simulink model "HSM_SMC_Final"  (R2018a)
settings: Solver=VariableStepAuto  StartTime=0.0  StopTime=0.1  RelTol=1e-3
InitFcn:
  | fsw = 20e3;
  | T = 1.0/fsw;
  | 
  | J=1.2e-7;
  | Pp = 50;
  | Ls=4.2e-3;
  | Rs=2.1;
  | Flux = 0.00425; %(Vs)
  | Km=Pp*Flux;
  | T_detent = 0.00065; %Nm
  | %------------------------------------
  | Ti=Ls/Rs;
  | rpmmax=200.0;
  | Tn = 2.0/100; %rated torque-Nm
  | TL = Tn;
  | Vdc = 24; %Vdc
  | umax=24; %dien ap cuc dai
  | imax=6; %dong cuc dai cua dong co
  | %------------------------------------
  | %Current controller
  | Kp_idq=0.5*umax/imax;
  | Ti_idq = Ls/Rs;
  | %Ti_idq = 0.009;
  | Ki_idq = Kp_idq/Ti_idq;
  | 
  | %Speed controller
  | Kp_Speed=imax/rpmmax;
  | Ti_Speed=0.25;
  | Ki_Speed = Kp_Speed/Ti_Speed;
  | T_spd = 1/1000;
  | 
  | %q axis maximum back EMF
  | EMFd_max  = (rpmmax/9.55)*Pp*Ls*imax;
  | Kp_Posision=rpmmax/(2*pi);
  | 
  | %ESO
  | fo = fsw/20;
  | %wo = 2*pi*fo;
  | wo = 200;
  | Beta1 = 2*wo;
  | Beta2 = wo*wo;
  | 
  | %Luenberger obs
  | K1 = 400;
  | K2 = 40000;
  | 
  | %PLL
  | kp = 6000;
  | ki = 60000;
  | 
  | %SMO
  | Ksw = 500;
  | wc = 2*pi*10;
undefined symbols (not defined in the file or in its folder): sigbuilder_block
libraries: powerlib x11, powerlib_meascontrol x1
settings Model: Creator=Admin  LastModifiedBy=DATPC
settings DataIOCC: ReturnWorkspaceOutputs=on
settings SFSimCC: SimUseLocalCustomCode=on
settings RTWCC: RTWUseLocalCustomCode=on

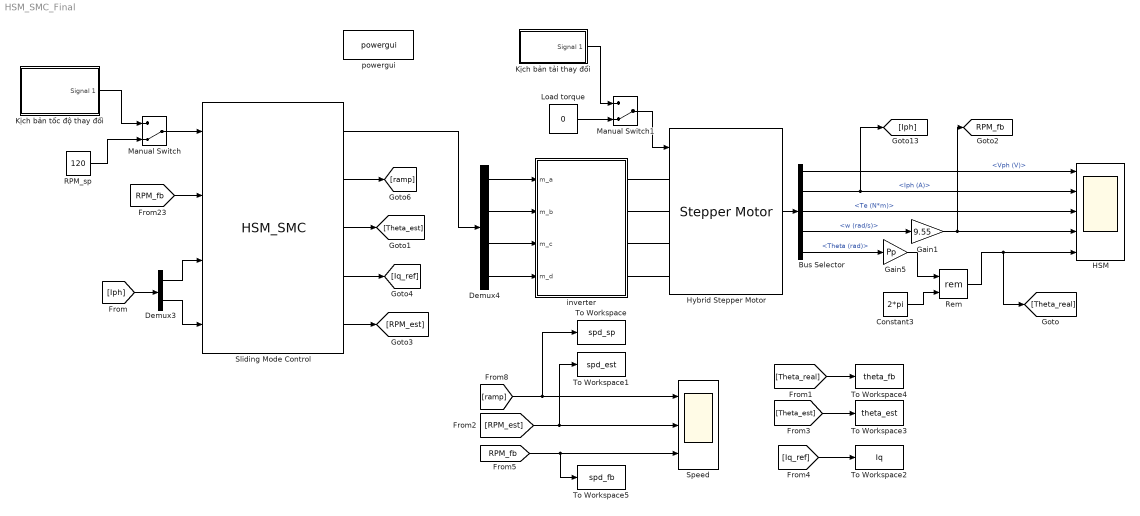
== system HSM_SMC_Final ==
  " Hybrid Stepper Motor" : powerlib/Machines/Stepper Motor  MotorType=Permanent-magnet / Hybrid  NumberOfPhases_1=2  NumberOfPhases_2=3  PresetModel_1=<empty>  PresetModel_2=<empty>  L=4.85e-3  Lmax=10e-3  Lmin=2e-3  R=2.5  Step_angle=1.8  Psim=0.00424  Tdm=0.00065  J=0.00058  B=0.0013  w0=0  pos0=0  TsPowergui=0  TsBlock=-1
      settings: SourceProductBaseCode=PS
  Bus Selector : BusSelector  OutputSignals=Vph (V),Iph (A),Te (N*m),w (rad/s),Theta (rad)
  Constant3 : Constant  Value=2*pi
  Demux3 : Demux  Outputs=2
  Demux4 : Demux
  Gain1 : Gain  Gain=9.55
  Gain5 : Gain  Gain=Pp
  "HSM " : Scope  NumInputPorts=5
  Kịch bản tải thay đổi : Subsystem  Tag=STV Subsys  LoadFcn=sigbuilder_block('load');  StartFcn=sigbuilder_block('start');  StopFcn=sigbuilder_block('stop');  ClipboardFcn=sigbuilder_block('clipboard');  mask(Sigbuilder block){tuvar=[0:10]}
      mask help: Simulink:masks:SigbuilderBlock_MD
      mask init:
      | if ~strcmp(get_param(bdroot(gcbh),'SimulationStatus'),'stopped') tuvar = sigbuilder_block('maskInit'); end
      settings: CopyFcn=sigbuilder_block('copy');  DeleteFcn=sigbuilder_block('delete');  ModelCloseFcn=sigbuilder_block('modelClose');  PreSaveFcn=sigbuilder_block('preSave');  PauseFcn=sigbuilder_block('pause');  ContinueFcn=sigbuilder_block('continue');  NameChangeFcn=sigbuilder_block('namechange');  OpenFcn=sigbuilder_block('open',[69.75 172.5 1141.5 477.75 ]);  CloseFcn=sigbuilder_block('close');
      mask Display: plot(0, 0, 100, 100,[2, 2, 32, 32, 2], [68, 8, 8, 68, 68],[32, 2], [38, 38], [32, 19, 2],[53, 60, 44], [32, 17, 17, 2],[16, 16, 31, 31]);txt = getActiveGroup(gcbh);text(2, 100, txt,'verticalAlignment', 'top');
  Kịch bản tốc độ thay đổi : Subsystem  Tag=STV Subsys  LoadFcn=sigbuilder_block('load');  StartFcn=sigbuilder_block('start');  StopFcn=sigbuilder_block('stop');  ClipboardFcn=sigbuilder_block('clipboard');  mask(Sigbuilder block){tuvar=[0:10]}
      mask help: Simulink:masks:SigbuilderBlock_MD
      mask init:
      | if ~strcmp(get_param(bdroot(gcbh),'SimulationStatus'),'stopped') tuvar = sigbuilder_block('maskInit'); end
      settings: CopyFcn=sigbuilder_block('copy');  DeleteFcn=sigbuilder_block('delete');  ModelCloseFcn=sigbuilder_block('modelClose');  PreSaveFcn=sigbuilder_block('preSave');  PauseFcn=sigbuilder_block('pause');  ContinueFcn=sigbuilder_block('continue');  NameChangeFcn=sigbuilder_block('namechange');  OpenFcn=sigbuilder_block('open',[6 30 1428 681.75 ]);  CloseFcn=sigbuilder_block('close');
      mask Display: plot(0, 0, 100, 100,[2, 2, 32, 32, 2], [68, 8, 8, 68, 68],[32, 2], [38, 38], [32, 19, 2],[53, 60, 44], [32, 17, 17, 2],[16, 16, 31, 31]);txt = getActiveGroup(gcbh);text(2, 100, txt,'verticalAlignment', 'top');
  Load torque : Constant  Value=0
  Manual Switch : ManualSwitch  CurrentSetting=0
  Manual Switch1 : ManualSwitch  CurrentSetting=0
  RPM_sp : Constant  Value=120
  Rem : Math  Operator=rem  SaturateOnIntegerOverflow=on
  Sliding Mode Control : S-Function  InitFcn=try, set_param(gcb,'FunctionName','HSM_SMC'), end  FunctionName=HSM_SMC  SFunctionModules=HSM_SMC_wrapper  SFunctionDeploymentMode=off  EnableBusSupport=off  mask(S-Function Builder){}
      mask help: Simulink:masks:SFunctionBuilder_MD
      mask init:
      | val = [[.9  0.75 0.75 1 1 .9 .9 1]',[1 1 0.75 0.75 .9 .9 1 .9]'];try , sys = get_param(gcb,'SfunBuilderFcnName');if isempty(sys), sys = get_param(gcb,'FunctionName'); end,catch, sys = get_param(gcb,'FunctionName'); end
      settings: CopyFcn=set_param(gcbh,'LinkStatus','none')  PreSaveFcn=try, set_param(gcb,'FunctionName','HSM_SMC'), end  OpenFcn=sfunctionwizard(gcbh)
      mask Display: plot(val(:,1),val(:,2)),disp(sys), port_label('input',1,'RPM_sp'), port_label('input',2,'RPM_fb'), port_label('input',3,'Ia_fb'), port_label('input',4,'Ib_fb'), port_label('output',1,'m'), port_label('output',2,'ramp'), port_label('output',3,'Theta_est'), port_label('output',4,'Iq_sp'), port_label('output',5,'RPM_est')
  Speed : Scope  NumInputPorts=3
  To Workspace : ToWorkspace  VariableName=spd_sp  SaveFormat=Timeseries  SampleTime=-1
  To Workspace1 : ToWorkspace  VariableName=spd_est  SaveFormat=Timeseries  SampleTime=-1
  To Workspace2 : ToWorkspace  VariableName=Iq  SaveFormat=Timeseries  SampleTime=-1
  To Workspace3 : ToWorkspace  VariableName=theta_est  SaveFormat=Timeseries  SampleTime=-1
  To Workspace4 : ToWorkspace  VariableName=theta_fb  SaveFormat=Timeseries  SampleTime=-1
  To Workspace5 : ToWorkspace  VariableName=spd_fb  SaveFormat=Timeseries  SampleTime=-1
  inverter : Subsystem
  powergui : powerlib/powergui  SimulationMode=Discrete  SampleTime=5e-8  frequency=60  Iterations=50  frequencyindice=0  Pbase=100e6  ErrMax=1e-4  UnitsV=kV  UnitsW=MW  buscounter=0  FunctionMessages=off  echomessages=off  EnableUseOfTLC=off  CurrentSourceSwitches=off  DisableSnubberDevices=off  DisableRonSwitches=off  DisableVfSwitches=off  DisplayEquations=off  SolverType=Tustin/Backward Euler (TBE)  Interpol=off  ExternalGateDelay=off  methode=off  Ts=100  x0status=blocks  SPID=off  SwTol=0  HookPort=off  RestoreLinks=warning  ResistiveCurrentMeasurement=off  Frange=[0:2:500]  Ylog=off  Xlog=on  ShowGrid=off  save=off  variable=ZData  structure=0  ZoomFFT=on  StartTime=0.0  cycles=1  DisplayStyle=1  fundamental=60  FreqAxis=off  MaxFrequency=1000  frequencyindicesteady=1  RmsSteady=1  display=off
  tag scope: RPM_fb=global
  wires:
  Bus Selector/2 -> "HSM "/2, [Iph]  "<Iph (A)>"
  Gain1/1 -> "HSM "/4, [RPM_fb]
  " Hybrid Stepper Motor"/1 -> Bus Selector/1
  Bus Selector/5 -> Gain5/1  "<Theta (rad)>"
  Bus Selector/1 -> "HSM "/1  "<Vph (V)>"
  Bus Selector/3 -> "HSM "/3  "<Te (N*m)>"
  Bus Selector/4 -> Gain1/1  "<w (rad/s)>"
  Demux3/1 -> Sliding Mode Control/3
  Demux3/2 -> Sliding Mode Control/4
  [Iph] -> Demux3/1
  Gain5/1 -> Rem/1
  Rem/1 -> [Theta_real], "HSM "/5
  [RPM_fb] -> Sliding Mode Control/2
  Demux4/1 -> inverter/1(m_a)
  Demux4/2 -> inverter/2(m_b)
  Demux4/3 -> inverter/3(m_c)
  Demux4/4 -> inverter/4(m_d)
  Sliding Mode Control/1 -> Demux4/1
  Manual Switch/1 -> Sliding Mode Control/1
  Constant3/1 -> Rem/2
  RPM_sp/1 -> Manual Switch/2
  Kịch bản tốc độ thay đổi/1(Signal 1) -> Manual Switch/1
  Manual Switch1/1 -> " Hybrid Stepper Motor"/1
  Load torque/1 -> Manual Switch1/2
  Kịch bản tải thay đổi/1(Signal 1) -> Manual Switch1/1
  Sliding Mode Control/5 -> [RPM_est]
  [RPM_est] -> To Workspace1/1, Speed/2
  Sliding Mode Control/2 -> [ramp]
  Sliding Mode Control/3 -> [Theta_est]
  Sliding Mode Control/4 -> [Iq_ref]
  [Iq_ref] -> To Workspace2/1
  [Theta_real] -> To Workspace4/1
  [Theta_est] -> To Workspace3/1
  [ramp] -> To Workspace/1, Speed/1
  [RPM_fb] -> To Workspace5/1, Speed/3
  connections:
  " Hybrid Stepper Motor"/LConn3 -- inverter/RConn3
  " Hybrid Stepper Motor"/LConn2 -- inverter/RConn2
  " Hybrid Stepper Motor"/LConn4 -- inverter/RConn4
  " Hybrid Stepper Motor"/LConn1 -- inverter/RConn1

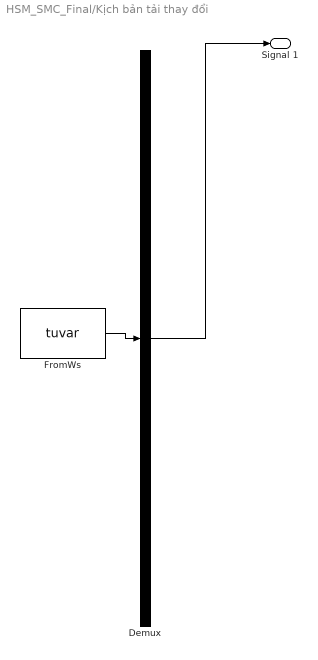
== system HSM_SMC_Final/Kịch bản tải thay đổi ==
  Demux : Demux  Tag=STV Demux  Outputs=1
  FromWs : FromWorkspace  Tag=STV FromWs  VariableName=tuvar  SampleTime=0
      SigBuilderData=|
      | common.afterFinalStr = 'Extrapolate'
      | common.sampleTime = 0
      | dataSet.timeRange = [0 1.5]
      | dataSet.name = 'Group 1'
      | sbobj.Groups.Name = 'Group 1'
      | sbobj.Groups.Signals.Name = 'Signal 1'
      | sbobj.Groups.Signals.XData = [0 0.4 0.4 1 1.5]
      | sbobj.Groups.Signals.YData = [0 0 0.02 0.02 0.02]
      | sbobj.Groups.TimeRange = [0 1.5]
  Signal 1 : Outport  Tag=STV Outport
  wires:
  Demux/1 -> Signal 1/1
  FromWs/1 -> Demux/1

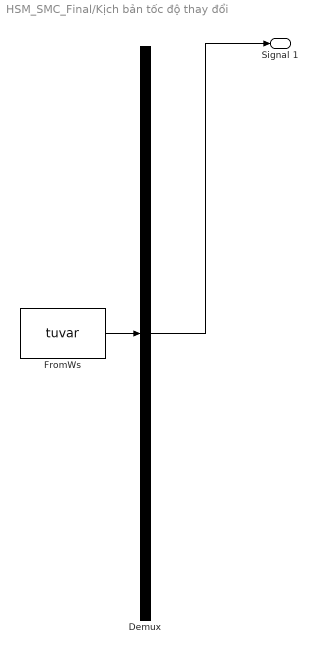
== system HSM_SMC_Final/Kịch bản tốc độ thay đổi ==
  Demux : Demux  Tag=STV Demux  Outputs=1
  FromWs : FromWorkspace  Tag=STV FromWs  VariableName=tuvar  SampleTime=0
      SigBuilderData=|
      | common.afterFinalStr = 'Extrapolate'
      | common.sampleTime = 0
      | dataSet.timeRange = [0 1.5]
      | dataSet.name = 'Group 1'
      | sbobj.Groups.Name = 'Group 1'
      | sbobj.Groups.Signals.Name = 'Signal 1'
      | sbobj.Groups.Signals.XData = [0 0.5 0.5 1 1 1.5]
      | sbobj.Groups.Signals.YData = [120 120 55 55 100 100]
      | sbobj.Groups.TimeRange = [0 1.5]
  Signal 1 : Outport  Tag=STV Outport
  wires:
  Demux/1 -> Signal 1/1
  FromWs/1 -> Demux/1

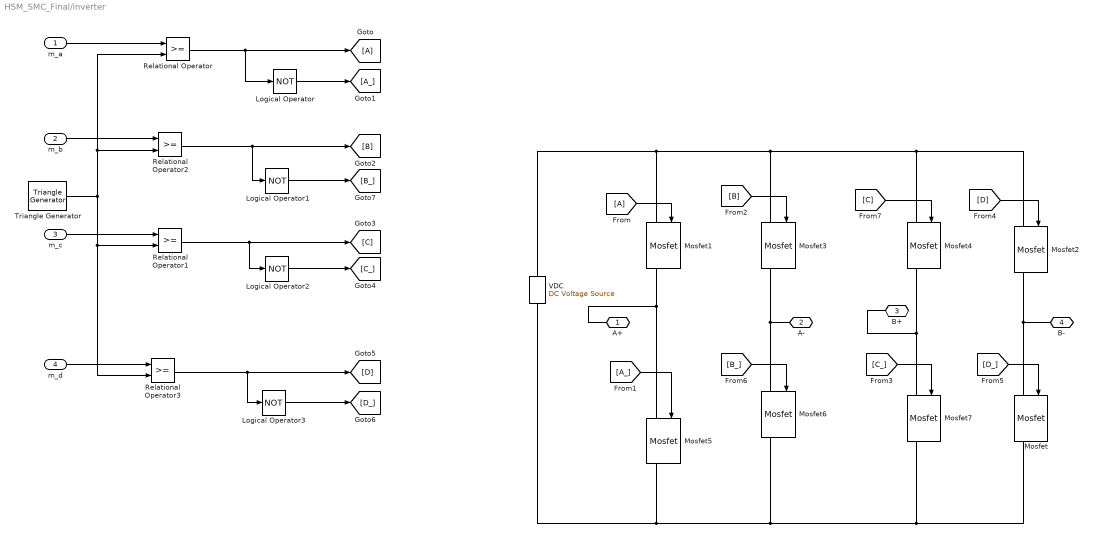
== system HSM_SMC_Final/inverter ==
  m_a : Inport
  m_b : Inport  Port=2
  m_c : Inport  Port=3
  m_d : Inport  Port=4
  Logical Operator{,1..3} (4 alike) : Logic  Operator=NOT  AllPortsSameDT=off  OutDataTypeStr=boolean
  Mosfet{,1..7} (8 alike) : powerlib/Power Electronics/Mosfet  Ron=0.1  Lon=0  Rd=0.01  Vfd=0  IC=0  Rs=1e5  Cs=inf  Measurements=on
  Relational Operator{,1..3} (4 alike) : RelationalOperator  OutDataTypeStr=boolean  RndMeth=Simplest
  Triangle Generator : powerlib_meascontrol/Pulse & Signal Generators/Triangle Generator  Freq=fsw  Phase=0  Ts=1e-8
  VDC : powerlib/Electrical Sources/DC Voltage Source  Amplitude=Vdc  Measurements=None
  A+ : PMIOPort  Side=Right
  A- : PMIOPort  Port=2  Side=Right
  B+ : PMIOPort  Port=3  Side=Right
  B- : PMIOPort  Port=4  Side=Right
  wires:
  Relational Operator/1 -> [A], Logical Operator/1
  Relational Operator2/1 -> Logical Operator1/1, [B]
  Logical Operator1/1 -> [B_]
  Relational Operator1/1 -> Logical Operator2/1, [C]
  Logical Operator2/1 -> [C_]
  Relational Operator3/1 -> Logical Operator3/1, [D]
  Logical Operator3/1 -> [D_]
  Logical Operator/1 -> [A_]
  [B] -> Mosfet3/1
  [B_] -> Mosfet6/1
  [D] -> Mosfet2/1
  [D_] -> Mosfet/1
  m_b/1 -> Relational Operator2/1
  m_c/1 -> Relational Operator1/1
  m_d/1 -> Relational Operator3/1
  [A] -> Mosfet1/1
  [A_] -> Mosfet5/1
  [C] -> Mosfet4/1
  [C_] -> Mosfet7/1
  m_a/1 -> Relational Operator/1
  Triangle Generator/1 -> Relational Operator3/2, Relational Operator1/2, Relational Operator2/2, Relational Operator/2
  connections:
  Mosfet3/RConn1 -- A-/RConn1 -- Mosfet6/LConn1
  Mosfet/LConn1 -- B-/RConn1 -- Mosfet2/RConn1
  Mosfet2/LConn1 -- Mosfet1/LConn1 -- VDC/RConn1 -- Mosfet3/LConn1 -- Mosfet4/LConn1
  Mosfet6/RConn1 -- Mosfet7/RConn1 -- Mosfet/RConn1 -- VDC/LConn1 -- Mosfet5/RConn1
  Mosfet1/RConn1 -- Mosfet5/LConn1 -- A+/RConn1
  Mosfet4/RConn1 -- Mosfet7/LConn1 -- B+/RConn1
